simulink model "promena_topologije_kontrolera_sim"  (R2020a)
settings: Solver=FixedStepAuto  StartTime=0.0  StopTime=sim_duration  FixedStep=1e-4  RelTol=1e-3
undefined symbols (not defined in the file): amp_poremecaj, amp_ref_stepdown1, amp_ref_stepdown2, amp_ref_stepup1, C, E, kontroler_pik, Kp, L, R, t_poremecaj, t_ref_stepdown1, t_ref_stepdown2, t_ref_stepup1, Td, Tf, Ti, Tt, ue, x2e
libraries: cstblocks x2
settings Model: Creator=HP  LastModifiedBy=HP

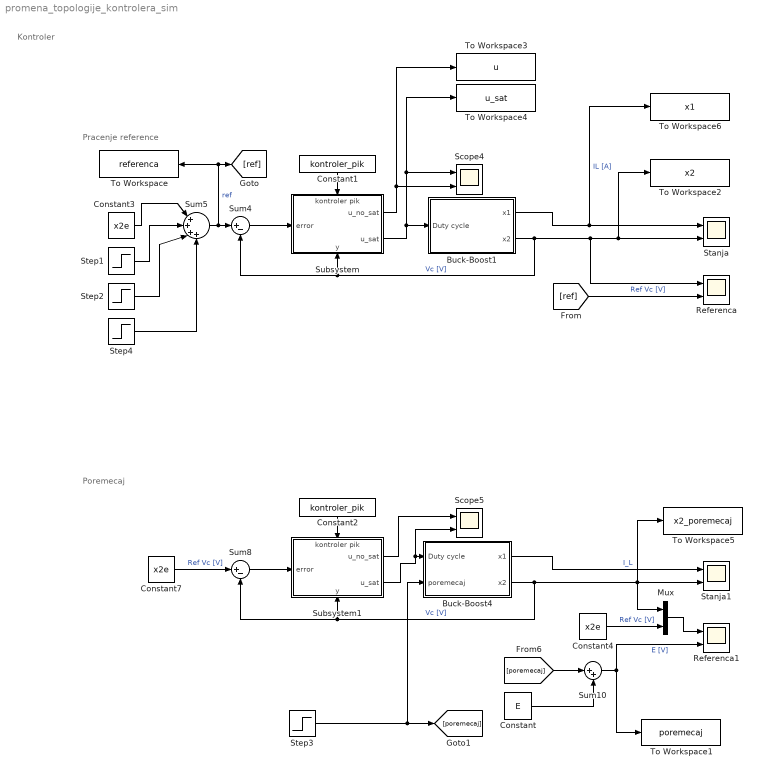
== system promena_topologije_kontrolera_sim ==
  note: Poremecaj
  note: Kontroler
  note: Pracenje reference
  Buck-Boost1 : Subsystem
  Buck-Boost4 : Subsystem
  Constant : Constant  Value=E
  Constant1 : Constant  Value=kontroler_pik
  Constant2 : Constant  Value=kontroler_pik
  Constant3 : Constant  Value=x2e
  Constant4 : Constant  Value=x2e
  Constant7 : Constant  Value=x2e
  Mux : Mux  Inputs=2
  Referenca : Scope  NumInputPorts=2
  Referenca1 : Scope  NumInputPorts=2
  Scope4 : Scope  NumInputPorts=2
  Scope5 : Scope  NumInputPorts=2
  Stanja : Scope  NumInputPorts=2
  Stanja1 : Scope  NumInputPorts=2
  Step1 : Step  Time=t_ref_stepdown1  After=amp_ref_stepdown1  SampleTime=0
  Step2 : Step  Time=t_ref_stepup1  After=amp_ref_stepup1  SampleTime=0
  Step3 : Step  Time=t_poremecaj  After=amp_poremecaj  SampleTime=0
  Step4 : Step  Time=t_ref_stepdown2  After=amp_ref_stepdown2  SampleTime=0
  Subsystem : Subsystem
      settings: PortSchema="{\"entries\":[{\"content\":{\"sides\":[{\"content\":{\"connectorIds\":[\"In1\"]},\"type\":\"ConnectorPlacement.EquallySpacedRectSide\",\"uuid\":\"0048fda4-5b4a-456a-8337-060e5808e354\"},{\"content\":{\"connectorIds\":[\"Out1\",\"Out2\"],\"side\":\"RIGHT\"},\"type\":\"ConnectorPlacement.EquallySpacedRectSide\",\"uuid\":\"02cdbfc3-6320-4e2f-beb2-fd4bcb343bc0\"},{\"content\":{\"connectorIds\":[\"In2\"],\"side\":\"TOP\"},\"type\":\"ConnectorPlacement.EquallySpacedRectSide\",\"uuid\":\"beb84629-8290-4bff-b476-a419e2f00711\"},{\"content\":{\"connectorIds\":[\"In3\"],\"side\":\"BOTTOM\"},\"type\":\"ConnectorPlacement.EquallySpacedRectSide\",\"uuid\":\"42e18825-4a79-44d0-8554-c303765f9505\"}]},\"type\":\"ConnectorPlacement.EquallySpacedConnector\",\"uuid\":\"e20d5ce2-d62d-498d-95ea-535548399f24\"}],\"packageUris\":[\"http://schema.mathworks.com/mf0/Connector/19700101\"],\"version\":\"1.0\"}"
  Subsystem1 : Subsystem
      settings: PortSchema="{\"entries\":[{\"content\":{\"sides\":[{\"content\":{\"connectorIds\":[\"In1\"]},\"type\":\"ConnectorPlacement.EquallySpacedRectSide\",\"uuid\":\"0048fda4-5b4a-456a-8337-060e5808e354\"},{\"content\":{\"connectorIds\":[\"Out1\",\"Out2\"],\"side\":\"RIGHT\"},\"type\":\"ConnectorPlacement.EquallySpacedRectSide\",\"uuid\":\"02cdbfc3-6320-4e2f-beb2-fd4bcb343bc0\"},{\"content\":{\"connectorIds\":[\"In2\"],\"side\":\"TOP\"},\"type\":\"ConnectorPlacement.EquallySpacedRectSide\",\"uuid\":\"beb84629-8290-4bff-b476-a419e2f00711\"},{\"content\":{\"connectorIds\":[\"In3\"],\"side\":\"BOTTOM\"},\"type\":\"ConnectorPlacement.EquallySpacedRectSide\",\"uuid\":\"42e18825-4a79-44d0-8554-c303765f9505\"}]},\"type\":\"ConnectorPlacement.EquallySpacedConnector\",\"uuid\":\"e20d5ce2-d62d-498d-95ea-535548399f24\"}],\"packageUris\":[\"http://schema.mathworks.com/mf0/Connector/19700101\"],\"version\":\"1.0\"}"
  Sum10 : Sum  Inputs=|++
  Sum4 : Sum  Inputs=|+-
  Sum5 : Sum  Inputs=|++++
  Sum8 : Sum  Inputs=|+-
  To Workspace : ToWorkspace  VariableName=referenca  SaveFormat=Timeseries  SampleTime=-1
  To Workspace1 : ToWorkspace  VariableName=poremecaj  SaveFormat=Timeseries  SampleTime=-1
  To Workspace2 : ToWorkspace  VariableName=x2  SaveFormat=Timeseries  SampleTime=-1
  To Workspace3 : ToWorkspace  VariableName=u  SaveFormat=Timeseries  SampleTime=-1
  To Workspace4 : ToWorkspace  VariableName=u_sat  SaveFormat=Timeseries  SampleTime=-1
  To Workspace5 : ToWorkspace  VariableName=x2_poremecaj  SaveFormat=Timeseries  SampleTime=-1
  To Workspace6 : ToWorkspace  VariableName=x1  SaveFormat=Timeseries  SampleTime=-1
  wires:
  Buck-Boost4/2(x2) -> To Workspace5/1, Mux/1, Stanja1/2, Subsystem1/3(y), Sum8/2  "Vc [V]"
  [ref] -> Referenca/2  "Ref Vc [V]"
  Step2/1 -> Sum5/3
  Buck-Boost4/1(x1) -> Stanja1/1  "I_L"
  Constant3/1 -> Sum5/1
  Constant/1 -> Sum10/2
  Constant7/1 -> Sum8/1  "Ref Vc [V]"
  [poremecaj] -> Sum10/1
  Buck-Boost1/2(x2) -> Referenca/1, To Workspace2/1, Stanja/2, Subsystem/3(y), Sum4/2  "Vc [V]"
  Mux/1 -> Referenca1/1
  Step1/1 -> Sum5/2
  Subsystem1/2(u_sat) -> Scope5/2, Buck-Boost4/1(Duty cycle)
  Sum5/1 -> Sum4/1, To Workspace/1, [ref]  "ref"
  Sum10/1 -> Referenca1/2, To Workspace1/1  "E [V]"
  Buck-Boost1/1(x1) -> To Workspace6/1, Stanja/1  "IL [A]"
  Step3/1 -> Buck-Boost4/2(poremecaj), [poremecaj]
  Step4/1 -> Sum5/4
  Constant1/1 -> Subsystem/2(kontroler pik)
  Constant2/1 -> Subsystem1/2(kontroler pik)
  Sum8/1 -> Subsystem1/1(error)
  Subsystem1/1(u_no_sat) -> Scope5/1
  Constant4/1 -> Mux/2  "Ref Vc [V]"
  Sum4/1 -> Subsystem/1(error)
  Subsystem/2(u_sat) -> Scope4/1, To Workspace4/1, Buck-Boost1/1(Duty cycle)
  Subsystem/1(u_no_sat) -> Scope4/2, To Workspace3/1

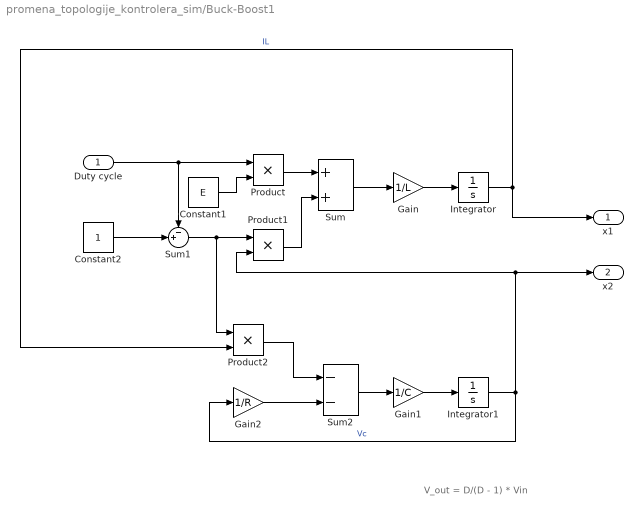
== system promena_topologije_kontrolera_sim/Buck-Boost1 ==
  note: V_out = D/(D - 1) * Vin
  Duty cycle : Inport
  Constant1 : Constant  Value=E
  Constant2 : Constant
  Gain : Gain  Gain=1/L
  Gain1 : Gain  Gain=1/C
  Gain2 : Gain  Gain=1/R
  Integrator : Integrator
  Integrator1 : Integrator
  Product : Product
  Product1 : Product
  Product2 : Product
  Sum : Sum
  Sum1 : Sum  Inputs=-+|
  Sum2 : Sum  Inputs=--
  x1 : Outport
  x2 : Outport  Port=2
  wires:
  Product/1 -> Sum/1
  Product1/1 -> Sum/2
  Sum2/1 -> Gain1/1
  Constant1/1 -> Product/2
  Integrator1/1 -> Gain2/1, x2/1, Product1/2  "Vc"
  Gain1/1 -> Integrator1/1
  Constant2/1 -> Sum1/2
  Integrator/1 -> x1/1, Product2/2  "IL"
  Sum/1 -> Gain/1
  Gain2/1 -> Sum2/2
  Sum1/1 -> Product2/1, Product1/1
  Duty cycle/1 -> Sum1/1, Product/1
  Product2/1 -> Sum2/1
  Gain/1 -> Integrator/1

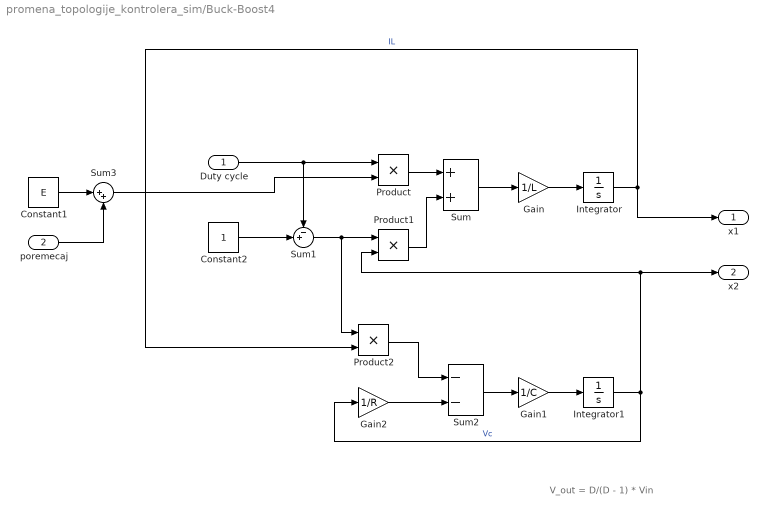
== system promena_topologije_kontrolera_sim/Buck-Boost4 ==
  note: V_out = D/(D - 1) * Vin
  Duty cycle : Inport
  poremecaj : Inport  Port=2
  Constant1 : Constant  Value=E
  Constant2 : Constant
  Gain : Gain  Gain=1/L
  Gain1 : Gain  Gain=1/C
  Gain2 : Gain  Gain=1/R
  Integrator : Integrator
  Integrator1 : Integrator
  Product : Product
  Product1 : Product
  Product2 : Product
  Sum : Sum
  Sum1 : Sum  Inputs=-+|
  Sum2 : Sum  Inputs=--
  Sum3 : Sum  Inputs=|++
  x1 : Outport
  x2 : Outport  Port=2
  wires:
  Product/1 -> Sum/1
  Product1/1 -> Sum/2
  Sum2/1 -> Gain1/1
  Integrator1/1 -> Gain2/1, x2/1, Product1/2  "Vc"
  Gain1/1 -> Integrator1/1
  Constant2/1 -> Sum1/2
  Integrator/1 -> x1/1, Product2/2  "IL"
  Sum/1 -> Gain/1
  Gain2/1 -> Sum2/2
  Sum1/1 -> Product2/1, Product1/1
  Duty cycle/1 -> Sum1/1, Product/1
  Product2/1 -> Sum2/1
  Gain/1 -> Integrator/1
  Constant1/1 -> Sum3/1
  Sum3/1 -> Product/2
  poremecaj/1 -> Sum3/2

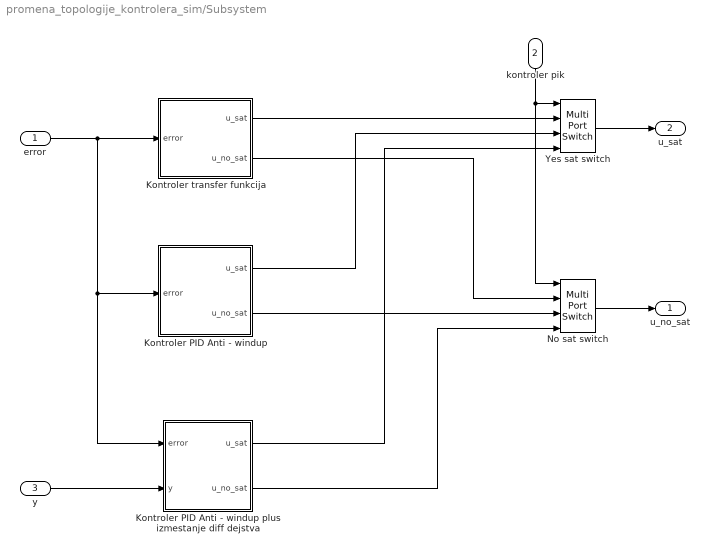
== system promena_topologije_kontrolera_sim/Subsystem ==
  error : Inport
  kontroler pik : Inport  Port=2
  y : Inport  Port=3
  Kontroler PID Anti - windup plus izmestanje diff dejstva : Subsystem
  Kontroler transfer funkcija : Subsystem
  Kontroler PID Anti - windup : Subsystem
  No sat switch : MultiPortSwitch
  Yes sat switch : MultiPortSwitch
  u_no_sat : Outport
  u_sat : Outport  Port=2
  wires:
  y/1 -> Kontroler PID Anti - windup plus izmestanje diff dejstva/2(y)
  Yes sat switch/1 -> u_sat/1
  kontroler pik/1 -> Yes sat switch/1, No sat switch/1
  error/1 -> Kontroler PID Anti - windup plus izmestanje diff dejstva/1(error), Kontroler PID Anti - windup/1(error), Kontroler transfer funkcija/1(error)
  Kontroler transfer funkcija/1(u_sat) -> Yes sat switch/2
  Kontroler PID Anti - windup plus izmestanje diff dejstva/2(u_no_sat) -> No sat switch/4
  Kontroler transfer funkcija/2(u_no_sat) -> No sat switch/2
  No sat switch/1 -> u_no_sat/1
  Kontroler PID Anti - windup plus izmestanje diff dejstva/1(u_sat) -> Yes sat switch/4
  Kontroler PID Anti - windup/2(u_no_sat) -> No sat switch/3
  Kontroler PID Anti - windup/1(u_sat) -> Yes sat switch/3

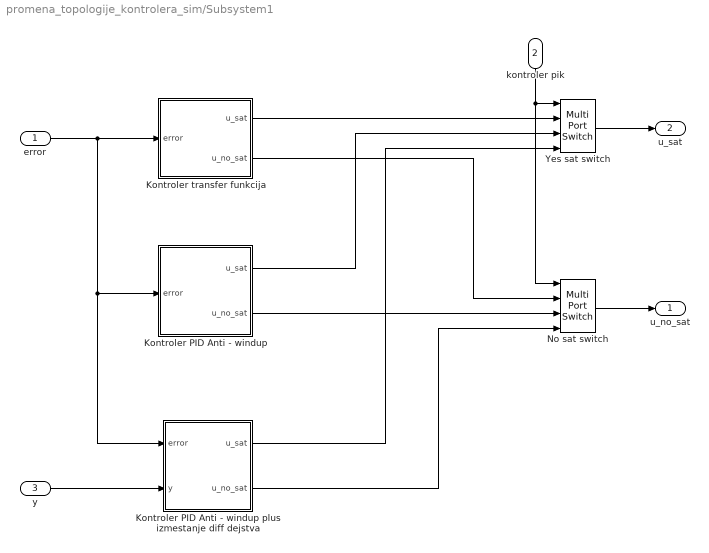
== system promena_topologije_kontrolera_sim/Subsystem1 ==
  error : Inport
  kontroler pik : Inport  Port=2
  y : Inport  Port=3
  Kontroler PID Anti - windup plus izmestanje diff dejstva : Subsystem
  Kontroler transfer funkcija : Subsystem
  Kontroler PID Anti - windup : Subsystem
  No sat switch : MultiPortSwitch
  Yes sat switch : MultiPortSwitch
  u_no_sat : Outport
  u_sat : Outport  Port=2
  wires:
  y/1 -> Kontroler PID Anti - windup plus izmestanje diff dejstva/2(y)
  Yes sat switch/1 -> u_sat/1
  kontroler pik/1 -> Yes sat switch/1, No sat switch/1
  error/1 -> Kontroler PID Anti - windup plus izmestanje diff dejstva/1(error), Kontroler PID Anti - windup/1(error), Kontroler transfer funkcija/1(error)
  Kontroler transfer funkcija/1(u_sat) -> Yes sat switch/2
  Kontroler PID Anti - windup plus izmestanje diff dejstva/2(u_no_sat) -> No sat switch/4
  Kontroler transfer funkcija/2(u_no_sat) -> No sat switch/2
  No sat switch/1 -> u_no_sat/1
  Kontroler PID Anti - windup plus izmestanje diff dejstva/1(u_sat) -> Yes sat switch/4
  Kontroler PID Anti - windup/2(u_no_sat) -> No sat switch/3
  Kontroler PID Anti - windup/1(u_sat) -> Yes sat switch/3

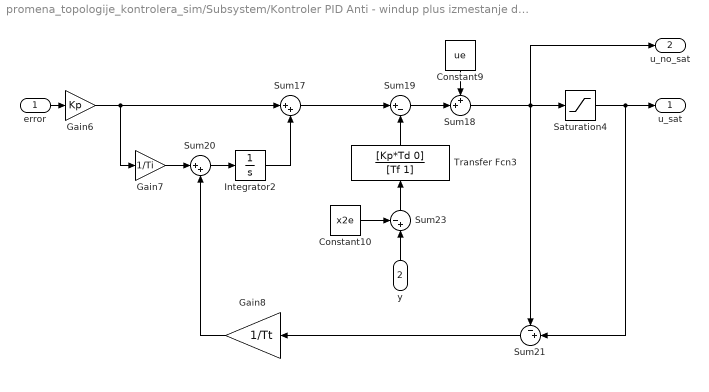
== system promena_topologije_kontrolera_sim/Subsystem/Kontroler PID Anti - windup plus izmestanje diff dejstva ==
  error : Inport
  y : Inport  Port=2
  Constant10 : Constant  Value=x2e
  Constant9 : Constant  Value=ue
  Gain6 : Gain  Gain=Kp
  Gain7 : Gain  Gain=1/Ti
  Gain8 : Gain  Gain=1/Tt
  Integrator2 : Integrator
  Saturation4 : Saturate  UpperLimit=1  LowerLimit=0
  Sum17 : Sum  Inputs=|++
  Sum18 : Sum  Inputs=++|
  Sum19 : Sum  Inputs=|+-
  Sum20 : Sum  Inputs=|++
  Sum21 : Sum  Inputs=-+|
  Sum23 : Sum  Inputs=-+|
  Transfer Fcn3 : TransferFcn  Numerator=[Kp*Td 0]  Denominator=[Tf 1]
  u_sat : Outport
  u_no_sat : Outport  Port=2
  wires:
  Transfer Fcn3/1 -> Sum19/2
  Sum18/1 -> Saturation4/1, u_no_sat/1, Sum21/1
  Integrator2/1 -> Sum17/2
  Sum17/1 -> Sum19/1
  error/1 -> Gain6/1
  y/1 -> Sum23/2
  Sum23/1 -> Transfer Fcn3/1
  Sum20/1 -> Integrator2/1
  Sum19/1 -> Sum18/2
  Constant9/1 -> Sum18/1
  Gain6/1 -> Sum17/1, Gain7/1
  Gain8/1 -> Sum20/2
  Gain7/1 -> Sum20/1
  Sum21/1 -> Gain8/1
  Constant10/1 -> Sum23/1
  Saturation4/1 -> Sum21/2, u_sat/1

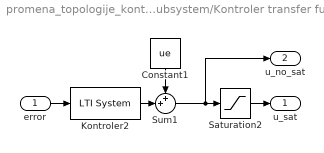
== system promena_topologije_kontrolera_sim/Subsystem/Kontroler transfer funkcija ==
  error : Inport
  Constant1 : Constant  Value=ue
  Kontroler2 : cstblocks/LTI System  sys=Kontroler  IC=[]
  Saturation2 : Saturate  UpperLimit=1  LowerLimit=0
  Sum1 : Sum  Inputs=++|
  u_sat : Outport
  u_no_sat : Outport  Port=2
  wires:
  Saturation2/1 -> u_sat/1
  Constant1/1 -> Sum1/1
  Sum1/1 -> u_no_sat/1, Saturation2/1
  Kontroler2/1 -> Sum1/2
  error/1 -> Kontroler2/1

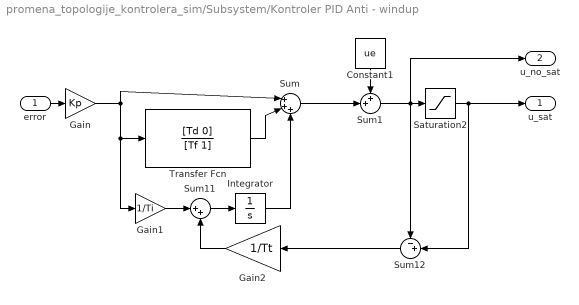
== system promena_topologije_kontrolera_sim/Subsystem/Kontroler PID Anti - windup ==
  error : Inport
  Constant1 : Constant  Value=ue
  Gain : Gain  Gain=Kp
  Gain1 : Gain  Gain=1/Ti
  Gain2 : Gain  Gain=1/Tt
  Integrator : Integrator
  Saturation2 : Saturate  UpperLimit=1  LowerLimit=0
  Sum : Sum  Inputs=|+++
  Sum1 : Sum  Inputs=++|
  Sum11 : Sum  Inputs=|++
  Sum12 : Sum  Inputs=-+|
  Transfer Fcn : TransferFcn  Numerator=[Td 0]  Denominator=[Tf 1]
  u_sat : Outport
  u_no_sat : Outport  Port=2
  wires:
  Integrator/1 -> Sum/3
  Sum11/1 -> Integrator/1
  Gain/1 -> Sum/1, Transfer Fcn/1, Gain1/1
  Sum1/1 -> u_no_sat/1, Sum12/1, Saturation2/1
  error/1 -> Gain/1
  Sum12/1 -> Gain2/1
  Saturation2/1 -> u_sat/1, Sum12/2
  Gain2/1 -> Sum11/2
  Constant1/1 -> Sum1/1
  Sum/1 -> Sum1/2
  Gain1/1 -> Sum11/1
  Transfer Fcn/1 -> Sum/2

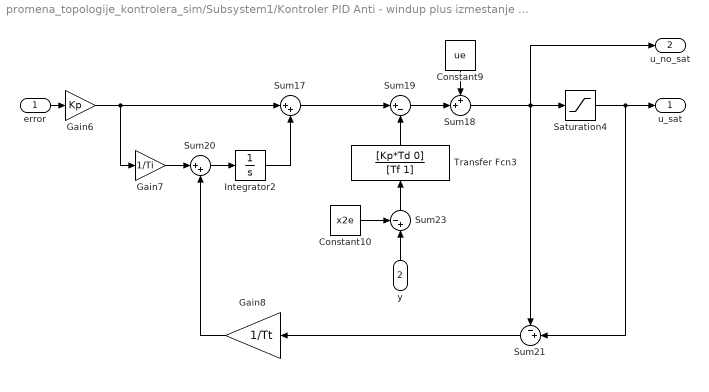
== system promena_topologije_kontrolera_sim/Subsystem1/Kontroler PID Anti - windup plus izmestanje diff dejstva ==
  error : Inport
  y : Inport  Port=2
  Constant10 : Constant  Value=x2e
  Constant9 : Constant  Value=ue
  Gain6 : Gain  Gain=Kp
  Gain7 : Gain  Gain=1/Ti
  Gain8 : Gain  Gain=1/Tt
  Integrator2 : Integrator
  Saturation4 : Saturate  UpperLimit=1  LowerLimit=0
  Sum17 : Sum  Inputs=|++
  Sum18 : Sum  Inputs=++|
  Sum19 : Sum  Inputs=|+-
  Sum20 : Sum  Inputs=|++
  Sum21 : Sum  Inputs=-+|
  Sum23 : Sum  Inputs=-+|
  Transfer Fcn3 : TransferFcn  Numerator=[Kp*Td 0]  Denominator=[Tf 1]
  u_sat : Outport
  u_no_sat : Outport  Port=2
  wires:
  Transfer Fcn3/1 -> Sum19/2
  Sum18/1 -> Saturation4/1, u_no_sat/1, Sum21/1
  Integrator2/1 -> Sum17/2
  Sum17/1 -> Sum19/1
  error/1 -> Gain6/1
  y/1 -> Sum23/2
  Sum23/1 -> Transfer Fcn3/1
  Sum20/1 -> Integrator2/1
  Sum19/1 -> Sum18/2
  Constant9/1 -> Sum18/1
  Gain6/1 -> Sum17/1, Gain7/1
  Gain8/1 -> Sum20/2
  Gain7/1 -> Sum20/1
  Sum21/1 -> Gain8/1
  Constant10/1 -> Sum23/1
  Saturation4/1 -> Sum21/2, u_sat/1

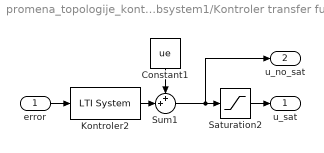
== system promena_topologije_kontrolera_sim/Subsystem1/Kontroler transfer funkcija ==
  error : Inport
  Constant1 : Constant  Value=ue
  Kontroler2 : cstblocks/LTI System  sys=Kontroler  IC=[]
  Saturation2 : Saturate  UpperLimit=1  LowerLimit=0
  Sum1 : Sum  Inputs=++|
  u_sat : Outport
  u_no_sat : Outport  Port=2
  wires:
  Saturation2/1 -> u_sat/1
  Constant1/1 -> Sum1/1
  Sum1/1 -> u_no_sat/1, Saturation2/1
  Kontroler2/1 -> Sum1/2
  error/1 -> Kontroler2/1

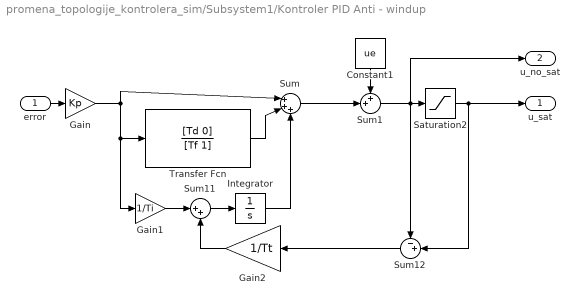
== system promena_topologije_kontrolera_sim/Subsystem1/Kontroler PID Anti - windup ==
  error : Inport
  Constant1 : Constant  Value=ue
  Gain : Gain  Gain=Kp
  Gain1 : Gain  Gain=1/Ti
  Gain2 : Gain  Gain=1/Tt
  Integrator : Integrator
  Saturation2 : Saturate  UpperLimit=1  LowerLimit=0
  Sum : Sum  Inputs=|+++
  Sum1 : Sum  Inputs=++|
  Sum11 : Sum  Inputs=|++
  Sum12 : Sum  Inputs=-+|
  Transfer Fcn : TransferFcn  Numerator=[Td 0]  Denominator=[Tf 1]
  u_sat : Outport
  u_no_sat : Outport  Port=2
  wires:
  Integrator/1 -> Sum/3
  Sum11/1 -> Integrator/1
  Gain/1 -> Sum/1, Transfer Fcn/1, Gain1/1
  Sum1/1 -> u_no_sat/1, Sum12/1, Saturation2/1
  error/1 -> Gain/1
  Sum12/1 -> Gain2/1
  Saturation2/1 -> u_sat/1, Sum12/2
  Gain2/1 -> Sum11/2
  Constant1/1 -> Sum1/1
  Sum/1 -> Sum1/2
  Gain1/1 -> Sum11/1
  Transfer Fcn/1 -> Sum/2
